simulink model "Darko"  (R2020b)
settings: Solver=VariableStepAuto  StartTime=0.0  StopTime=10.0  RelTol=1e-3
values from neighbouring files (symbols this model uses):
  initial_state = [p_initial; v_initial; omega_initial; q_initial]    [run.m]
  initial_state2 = [v_initial; omega_initial; q_initial]    [run.m]
libraries: sharedtransform x1
settings Model: Creator=florian  LastModifiedBy=florian

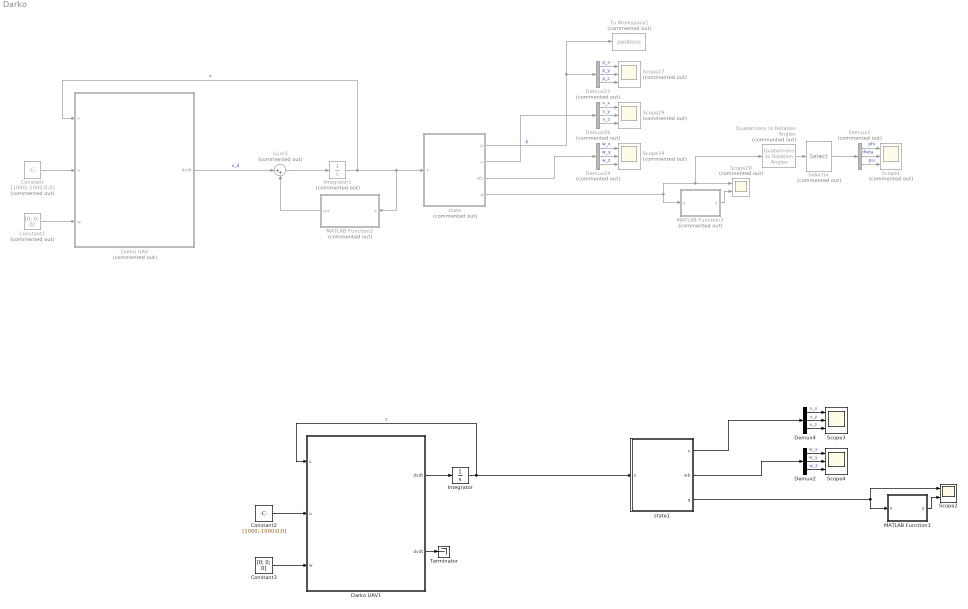
== system Darko ==
  Constant : Constant  Commented=on  Value=[1000;-1000;0;0]
  Constant1 : Constant  Commented=on  Value=[0; 0; 0]
  Constant2 : Constant  Value=[1000;-1000;0;0]
  Constant3 : Constant  Value=[0; 0; 0]
  Darko UAV : MATLAB Function  Commented=on  TreatAsAtomicUnit=on
  Darko UAV1 : MATLAB Function  TreatAsAtomicUnit=on
  Demux{1,24..26} (4 alike) : Demux  Commented=on  Outputs=3
  Demux2 : Demux  Outputs=3
  Demux4 : Demux  Outputs=3
  Integrator : Integrator  InitialCondition=initial_state2
  Integrator1 : Integrator  Commented=on  InitialCondition=initial_state
  MATLAB Function1 : MATLAB Function  TreatAsAtomicUnit=on
  MATLAB Function2 : MATLAB Function  Commented=on  TreatAsAtomicUnit=on
  MATLAB Function3 : MATLAB Function  Commented=on  TreatAsAtomicUnit=on
  Quaternions to Rotation Angles : sharedtransform/Quaternions to Rotation Angles  Commented=on  rotationOrder=ZXY  aMode=aMode
      settings: SourceProductBaseCode=AE,PW,MT,UV,VE,VP
  Scope{1,27,29,34} (4 alike) : Scope  Commented=on  NumInputPorts=3
  Scope2 : Scope  NumInputPorts=2
  Scope28 : Scope  Commented=on  NumInputPorts=2
  Scope3 : Scope  NumInputPorts=3
  Scope4 : Scope  NumInputPorts=3
  Selector : Selector  Commented=on  InputPortWidth=3  IndexOptions=Index vector (dialog)  Indices=[2 3 1]  OutputSizes=1
  Sum5 : Sum  Commented=on  Inputs=|++
  Terminator : Terminator
  To Workspace1 : ToWorkspace  Commented=on  VariableName=positions  SampleTime=-1
  state : MATLAB Function  Commented=on  TreatAsAtomicUnit=on
  state1 : MATLAB Function  TreatAsAtomicUnit=on
  wires:
  Sum5/1 -> Integrator1/1
  Constant/1 -> Darko UAV/2(u)
  Constant1/1 -> Darko UAV/3(w)
  MATLAB Function2/1(cor) -> Sum5/2
  Darko UAV/1(dxdt) -> Sum5/1  "x_d"
  Integrator1/1 -> state/1(x), MATLAB Function2/1(x), Darko UAV/1(x)  "x"
  Demux1/3 -> Scope1/3  "psi"
  Selector/1 -> Demux1/1
  Demux26/3 -> Scope29/3  "v_z"
  Demux26/2 -> Scope29/2  "v_y"
  Demux24/1 -> Scope34/1  "w_x"
  state/2(v) -> Demux26/1
  MATLAB Function3/1(y) -> Scope28/2
  Demux24/3 -> Scope34/3  "w_z"
  Quaternions to Rotation Angles/1 -> Selector/1
  Demux1/2 -> Scope1/2  "theta"
  state/3(wb) -> Demux24/1
  Demux1/1 -> Scope1/1  "phi"
  Demux24/2 -> Scope34/2  "w_y"
  state/4(q) -> Quaternions to Rotation Angles/1, Scope28/1, MATLAB Function3/1(u)
  Demux26/1 -> Scope29/1  "v_x"
  state/1(p) -> To Workspace1/1, Demux25/1  "p"
  Demux25/2 -> Scope27/2  "p_y"
  Demux25/3 -> Scope27/3  "p_z"
  Demux25/1 -> Scope27/1  "p_x"
  Darko UAV1/2(dvdt) -> Terminator/1
  Constant3/1 -> Darko UAV1/3(w)
  Constant2/1 -> Darko UAV1/2(u)
  Demux2/1 -> Scope4/1  "w_x"
  state1/2(wb) -> Demux2/1
  Integrator/1 -> Darko UAV1/1(x), state1/1(x)  "x"
  Demux4/2 -> Scope3/2  "v_y"
  Demux4/3 -> Scope3/3  "v_z"
  state1/1(v) -> Demux4/1
  Demux2/3 -> Scope4/3  "w_z"
  Demux4/1 -> Scope3/1  "v_x"
  Demux2/2 -> Scope4/2  "w_y"
  MATLAB Function1/1(y) -> Scope2/2
  state1/3(q) -> Scope2/1, MATLAB Function1/1(u)
  Darko UAV1/1(dxdt) -> Integrator/1

== matlab function Darko/Darko UAV ==
  data: x input; u input; dxdt output; w input; drone parameter
function dxdt  = fcn(x, u, w, drone)
%#codegen

dxdt = sysEqt(x, u, w, drone);

== matlab function Darko/Darko UAV1 ==
  data: x input; u input; dxdt output; w input; dvdt output; drone parameter
function [dxdt, dvdt] = fcn(x, u, w, drone)
dxdt = sysEqt_origin(x, u, w, drone);
dvdt = dxdt(1:3);

== matlab function Darko/state1 ==
  data: x input; v output; wb output; q output
function [v, wb, q] = demux(x)
%#codegen


v = x(1:3);
wb = x(4:6);
q  = x(7:10);
% p_v = x(1:6);
% q_omega = [q; wb];

== matlab function Darko/MATLAB Function1 ==
  data: u input; y output
function y = fcn(u)
%#codegen

y = norm(u);

== matlab function Darko/MATLAB Function2 ==
  data: x input; cor output
function cor  = fcn(x)
%#codegen
q  = x(10:13);
n = norm(q);
mismatch = 1-n;
cor = [0;0;0; 0;0;0; 0;0;0; mismatch*q];

== matlab function Darko/MATLAB Function3 ==
  data: u input; y output
function y = fcn(u)
%#codegen

y = norm(u);

== matlab function Darko/state ==
  data: x input; p output; v output; wb output; q output
function [p, v, wb, q] = demux(x)
%#codegen

p = x(1:3);
v = x(4:6);
wb = x(7:9);
q  = x(10:13);
% p_v = x(1:6);
% q_omega = [q; wb];
